simulink model "ode2"  (Simulink 8.0)
settings: Solver=ode4  StartTime=0.0  StopTime=10.0  FixedStep=0.01  RelTol=1e-3
libraries: simulink x1
settings Model: Creator=CAD  LastModifiedBy=CAD

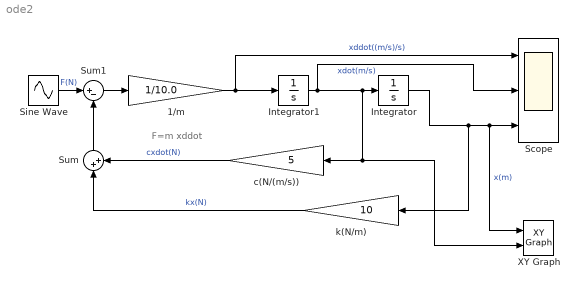
== system ode2 ==
  note: F=m xddot
  1/m : Gain  Gain=1/10.0
  Integrator : Integrator  InitialCondition=5
  Integrator1 : Integrator
  Scope : Scope  NumInputPorts=3
      settings: TimeRange=10  YMin=-5~-5~-5  YMax=5~5~5
  Sine Wave : Sin  Amplitude=0  SampleTime=0
  Sum : Sum  Inputs=|++
  Sum1 : Sum  Inputs=|+-
  XY Graph : simulink/Sinks/XY Graph  xmin=-6  xmax=6  ymin=-6  ymax=6  st=-1
  c(N/(m/s)) : Gain  Gain=5
  k(N/m) : Gain  Gain=10
  wires:
  1/m/1 -> Scope/1, Integrator1/1  "xddot((m/s)/s)"
  Integrator/1 -> k(N/m)/1, XY Graph/1, Scope/3  "x(m)"
  Integrator1/1 -> Scope/2, XY Graph/2, c(N/(m/s))/1, Integrator/1  "xdot(m/s)"
  k(N/m)/1 -> Sum/1  "kx(N)"
  c(N/(m/s))/1 -> Sum/2  "cxdot(N)"
  Sum1/1 -> 1/m/1
  Sine Wave/1 -> Sum1/1  "F(N)"
  Sum/1 -> Sum1/2
